simulink library "getCP_ul"  (R2020a)
settings: Solver=VariableStepAuto  StartTime=0.0  StopTime=10.0  RelTol=1e-3
undefined symbols (not defined in the file): Veh
settings Model: Creator=John Jr  LastModifiedBy=John Jr

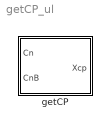
== system getCP_ul ==
  getCP : Subsystem

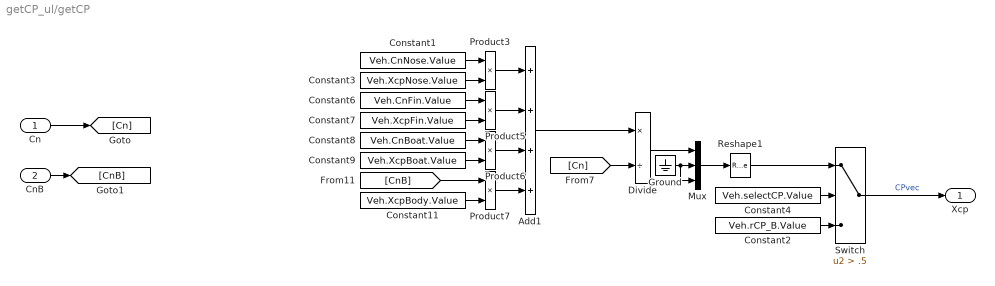
== system getCP_ul/getCP ==
  Cn : Inport
  CnB : Inport  Port=2
  Add1 : Sum  Inputs=++++
  Constant1 : Constant  Value=Veh.CnNose.Value
  Constant11 : Constant  Value=Veh.XcpBody.Value
  Constant2 : Constant  Value=Veh.rCP_B.Value
  Constant3 : Constant  Value=Veh.XcpNose.Value
  Constant4 : Constant  Value=Veh.selectCP.Value
  Constant6 : Constant  Value=Veh.CnFin.Value
  Constant7 : Constant  Value=Veh.XcpFin.Value
  Constant8 : Constant  Value=Veh.CnBoat.Value
  Constant9 : Constant  Value=Veh.XcpBoat.Value
  Divide : Product  Inputs=*/
  Ground : Ground
  Mux : Mux  Inputs=3
  Product{3,5..7} (4 alike) : Product
  Reshape1 : Reshape  OutputDimensionality=Column vector (2-D)
  Switch : Switch  Criteria=u2 > Threshold  Threshold=.5
  Xcp : Outport
  wires:
  Constant4/1 -> Switch/2
  Switch/1 -> Xcp/1  "CPvec"
  Reshape1/1 -> Switch/1
  Constant2/1 -> Switch/3
  Mux/1 -> Reshape1/1
  Ground/1 -> Mux/2, Mux/3
  Divide/1 -> Mux/1
  CnB/1 -> [CnB]
  Cn/1 -> [Cn]
  Product6/1 -> Add1/3
  [CnB] -> Product7/1
  Constant1/1 -> Product3/1
  Constant7/1 -> Product5/2
  Add1/1 -> Divide/1
  Constant6/1 -> Product5/1
  Product7/1 -> Add1/4
  [Cn] -> Divide/2
  Constant9/1 -> Product6/2
  Constant11/1 -> Product7/2
  Product5/1 -> Add1/2
  Constant8/1 -> Product6/1
  Constant3/1 -> Product3/2
  Product3/1 -> Add1/1
